simulink model "Battery_v3"  (R2024b)
settings: Solver=VariableStepAuto  StartTime=0.0  StopTime=inf  RelTol=1e-3
settings Model: Creator=miche  LastModifiedBy=miche

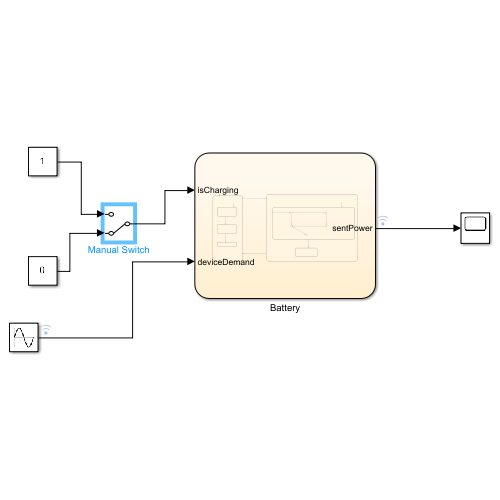
[thumbnail: Simulink's stored preview of the top-level diagram]
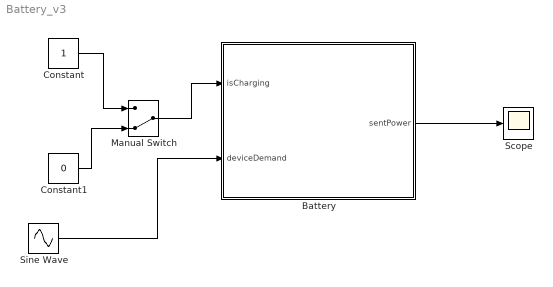
== system Battery_v3 ==
  Battery : Stateflow chart  TreatAsAtomicUnit=on
  Constant : Constant  SampleTime=0.5
  Constant1 : Constant  Value=0  SampleTime=0.5
  Manual Switch : ManualSwitch  CurrentSetting=0
  Scope : Scope
  Sine Wave : Sin  Amplitude=2.5  Bias=2.5  Phase=-pi/4  SampleTime=0
  wires:
  Constant/1 -> Manual Switch/1
  Constant1/1 -> Manual Switch/2
  Manual Switch/1 -> Battery/1(isCharging)
  Battery/1(sentPower) -> Scope/1
  Sine Wave/1 -> Battery/2(deviceDemand)

== stateflow chart Battery_v3/Battery ==
  state Discharge
    state Powered
      Powered -> (junction 19) [order 1]
      (junction 19) -> (junction 20) [order 1] : [deviceDemand>maxPower]
      (junction 19) -> (junction 24) [order 2] : {sentPower = deviceDemand;}
      (junction 20) -> (junction 21) : {sentPower = maxPower;}
      (junction 21) -> (junction 24)
      (junction 24) -> (junction 27) : {charge = charge - sentPower; }
    state Empty
      entry:
      sentPower = 0;
    (default) -> Powered
    Powered -> Empty [order 1] : [charge<=3]
  state Charge
    entry:
    sentPower = 0;
    state FastCharge
      during:
      charge = charge +4;
    state SlowChart
      during:
      charge = charge +1
    state Full
    (default) -> FastCharge
    FastCharge -> SlowChart : [charge > 80]
    SlowChart -> Full : [charge == 100]
  (default) -> Charge
  Charge -> Discharge : [~isCharging]
  Discharge -> Charge : [isCharging]
  data: isCharging input; sentPower output; charge local =50; maxPower local =3.5; deviceDemand input
